simulink model "sim_pendulum_v02"  (R2025b)
settings: Solver=FixedStepAuto  StartTime=0.0  StopTime=30  FixedStep=Ts  RelTol=1e-6
values from neighbouring files (symbols this model uses):
  pendulum = Pendulum()    [KF_EKF_SIM_TEST.m]    (also in nss_pendulum_sim.m; nss_pendulum_sim_dynamicchar.m = sys; nss_pendulum_sim_staticchar.m = sys)
  R = 0.01    [KF_EKF_SIM_TEST.m]    (also in nss_pendulum_sim.m = 0.000225; sim_main.m; simulate_sys.m = ones(1, 1); simulate_sys_ekf.m = ones(1, 1))
  Ts = 0.05    [KF_EKF_SIM_TEST.m]    (also in nss_pendulum_sim.m = 0.1; nss_pendulum_sim_dynamicchar.m; nss_pendulum_sim_staticchar.m; sim_main.m = 0.02)
undefined symbols (not defined in the file or in its folder): A, B, C, Discrete, Time
libraries: simulink_extras x2, ctrlSharedLib x1
settings Model: Creator=rjrad  LastModifiedBy=rjrad
settings DataIOCC: SaveOutput=off  DSMLogging=off  SaveTime=off  ReturnWorkspaceOutputs=off

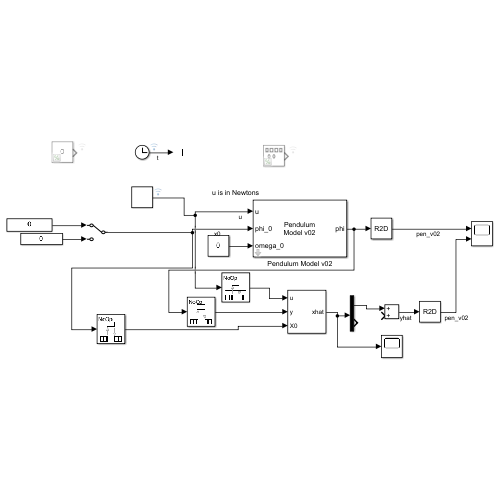
[thumbnail: Simulink's stored preview of the top-level diagram]
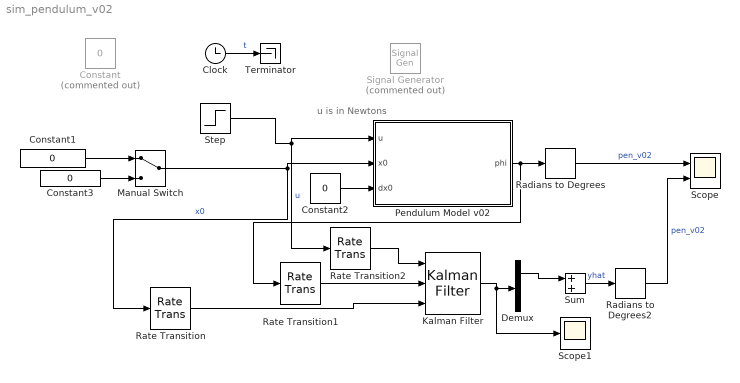
== system sim_pendulum_v02 ==
  note: u is in Newtons
  Clock : Clock
  Constant : Constant  Commented=on  Value=0
  Constant1 : Constant  Value=0
  Constant2 : Constant  Value=0
  Constant3 : Constant  Value=0
  Demux : Demux  Outputs=2
  Kalman Filter : ctrlSharedLib/Kalman Filter  TimeDomain=Discrete-Time  UseCurrentEstimator=on  ModelSource=Individual A, B, C, D matrices  ModelSourceVariable=ss(0.95,1,1,0,1)  A=A  B=B  C=C  D=0  NumberOfStates=1  NumberOfInputs=1  NumberOfOutputs=1  InitialEstimateSource=Input port  X0=0  P0=10  UseK=off  UseGH=off  NumberOfProcessNoiseInputs=1  G=1  TimeInvariantG=on  H=0  TimeInvariantH=on  Q=Q  TimeInvariantQ=on  R=R  TimeInvariantR=on  N=0  TimeInvariantN=on  AddInputPort=on  AddEnablePort=off  OutputEstimatedY=off  OutputP=off  Ts=-1
  Manual Switch : ManualSwitch
  Pendulum Model v02 : Subsystem  mask{pendulum=pendulum, sim_friction=on}
      mask prompts: sim_friction "Simulate friction?"
      mask DialogControl sim_opts Prompt: Simulation options
      mask Display:
      | disp('Pendulum\nModel v02');
      | port_label('output', 1, 'phi');
      | port_label('input', 1, 'u');
      | port_label('input', 2, 'phi_0');
      | port_label('input', 3, 'omega_0');
  Radians to Degrees : simulink_extras/Transformations/Radians to Degrees
  Radians to Degrees2 : simulink_extras/Transformations/Radians to Degrees
  Rate Transition : RateTransition  OutPortSampleTime=Ts
  Rate Transition1 : RateTransition  OutPortSampleTime=Ts
  Rate Transition2 : RateTransition  OutPortSampleTime=Ts
  Scope : Scope  NumInputPorts=2
      settings: ActiveDisplayYMinimum=-54.483516065587629  ActiveDisplayYMaximum=58.132748337938317
  Scope1 : Scope
      settings: ActiveDisplayYMinimum=-6.1993384412738113  ActiveDisplayYMaximum=5.9572861302206661  DataLoggingVariableName=ScopeData2
  Signal Generator : SignalGenerator  Commented=on  WaveForm=sawtooth  Frequency=0.1
  Step : Step  Time=Ts  Before=100  After=0  SampleTime=0
  Sum : Sum
  Terminator : Terminator
  wires:
  Radians to Degrees/1 -> Scope/1  "pen_v02"
  Clock/1 -> Terminator/1  "t"
  Step/1 -> Pendulum Model v02/1(u), Rate Transition2/1  "u"
  Pendulum Model v02/1(phi) -> Rate Transition1/1, Radians to Degrees/1
  Constant3/1 -> Manual Switch/2
  Constant1/1 -> Manual Switch/1
  Constant2/1 -> Pendulum Model v02/3(dx0)
  Manual Switch/1 -> Rate Transition/1, Pendulum Model v02/2(x0)  "x0"
  Kalman Filter/1 -> Scope1/1, Demux/1
  Demux/1 -> Sum/1
  Sum/1 -> Radians to Degrees2/1  "yhat"
  Rate Transition/1 -> Kalman Filter/3
  Rate Transition1/1 -> Kalman Filter/2
  Rate Transition2/1 -> Kalman Filter/1
  Radians to Degrees2/1 -> Scope/2  "pen_v02"

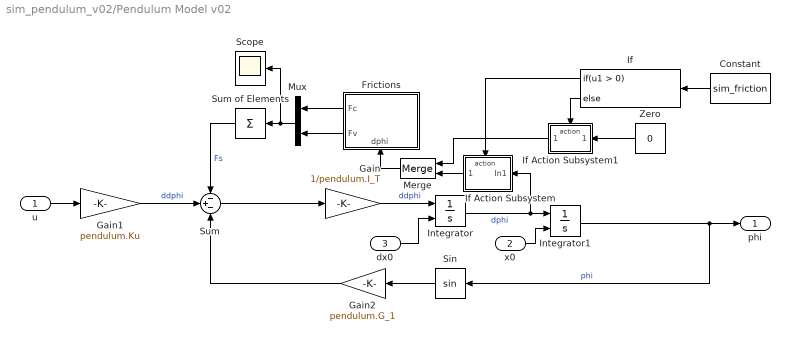
== system sim_pendulum_v02/Pendulum Model v02 ==
  u : Inport
  x0 : Inport  Port=2
  dx0 : Inport  Port=3
  Constant : Constant  Value=sim_friction
  Frictions : Subsystem
      settings: PortSchema="{\"entries\":[{\"content\":{\"sides\":[{\"content\":{},\"type\":\"ConnectorPlacement.EquallySpacedRectSide\",\"uuid\":\"0e17ee99-558a-4b29-b1de-7b93a8b61d87\"},{\"content\":{\"connectorIds\":[\"Out1\",\"Out2\"],\"side\":\"RIGHT\"},\"type\":\"ConnectorPlacement.EquallySpacedRectSide\",\"uuid\":\"5e5caba9-03ca-471d-81cf-f8a9a96e4230\"},{\"content\":{\"side\":\"TOP\"},\"type\":\"ConnectorPlacement.EquallySpacedRectSide\",\"uuid\":\"96b5fe86-242a-4b22-b30c-8698f3707795\"},{\"content\":{\"connectorIds\":[\"In1\"],\"side\":\"BOTTOM\"},\"type\":\"ConnectorPlacement.EquallySpacedRectSide\",\"uuid\":\"1ddafc32-a5e2-48b5-ab8a-03e3da860299\"}]},\"type\":\"ConnectorPlacement.EquallySpacedConnector\",\"uuid\":\"6166b7f2-3467-4650-975d-bbc4e263d57b\"}],\"packageUris\":[\"http://schema.mathworks.com/mf0/Connector/R2020b\"],\"version\":\"1.0\"}"
  Gain : Gain  Gain=1/pendulum.I_T
  Gain1 : Gain  Gain=pendulum.Ku
  Gain2 : Gain  Gain=pendulum.G_1
  If : If
  If Action Subsystem : Subsystem  TreatAsAtomicUnit=on
  If Action Subsystem1 : Subsystem  TreatAsAtomicUnit=on
  Integrator : Integrator  InitialConditionSource=external
  Integrator1 : Integrator  InitialConditionSource=external
  Merge : Merge
  Mux : Mux  Inputs=2
  Scope : Scope
      settings: ActiveDisplayYMinimum=-0.00069957503919249313  ActiveDisplayYMaximum=0.00072534349590993241
  Sin : Trigonometry
  Sum : Sum  Inputs=-+-
  Sum of Elements : Sum  Inputs=+
  Zero : Constant  Value=0  OutDataTypeStr=Inherit: Inherit via back propagation
  phi : Outport
  wires:
  Integrator1/1 -> phi/1, Sin/1  "phi"
  Gain/1 -> Integrator/1  "ddphi"
  Sin/1 -> Gain2/1
  Integrator/1 -> If Action Subsystem/1(In1), Integrator1/1  "dphi"
  Gain2/1 -> Sum/3
  Sum/1 -> Gain/1
  dx0/1 -> Integrator/2
  x0/1 -> Integrator1/2
  u/1 -> Gain1/1
  Sum of Elements/1 -> Sum/1  "Fs"
  Frictions/1(Fc) -> Mux/1
  Frictions/2(Fv) -> Mux/2
  Mux/1 -> Scope/1, Sum of Elements/1
  Constant/1 -> If/1
  Merge/1 -> Frictions/1(dphi)
  If Action Subsystem/1(Out1) -> Merge/2
  Zero/1 -> If Action Subsystem1/1(In1)
  If/1 -> If Action Subsystem/Action
  If Action Subsystem1/1(Out1) -> Merge/1
  If/2 -> If Action Subsystem1/Action
  Gain1/1 -> Sum/2  "ddphi"

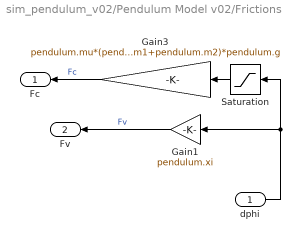
== system sim_pendulum_v02/Pendulum Model v02/Frictions ==
  dphi : Inport
  Gain1 : Gain  Gain=pendulum.xi
  Gain3 : Gain  Gain=pendulum.mu*(pendulum.m1+pendulum.m2)*pendulum.g
  Saturation : Saturate  UpperLimit=1  LowerLimit=-1
  Fc : Outport
  Fv : Outport  Port=2
  wires:
  dphi/1 -> Saturation/1, Gain1/1
  Gain3/1 -> Fc/1  "Fc"
  Saturation/1 -> Gain3/1
  Gain1/1 -> Fv/1  "Fv"

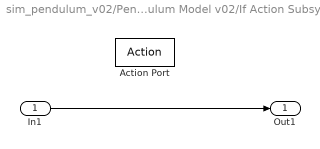
== system sim_pendulum_v02/Pendulum Model v02/If Action Subsystem ==
  In1 : Inport
  Action Port : ActionPort  ActionPortLabel=if(u1 > 0)
  Out1 : Outport
  wires:
  In1/1 -> Out1/1

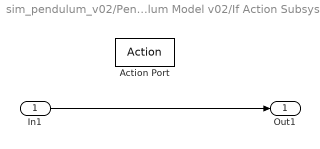
== system sim_pendulum_v02/Pendulum Model v02/If Action Subsystem1 ==
  In1 : Inport
  Action Port : ActionPort  ActionPortLabel=else
  Out1 : Outport
  wires:
  In1/1 -> Out1/1
